simulink model "Test_of_GeneralForceCtro_VBS_Controller_tau_w"  (R2023a)
settings: Solver=FixedStepAuto  StartTime=0.0  StopTime=150  FixedStep=0.0001  RelTol=1e-3
libraries: simulink x2
settings Model: Creator=邓宇飞  LastModifiedBy=邓宇飞

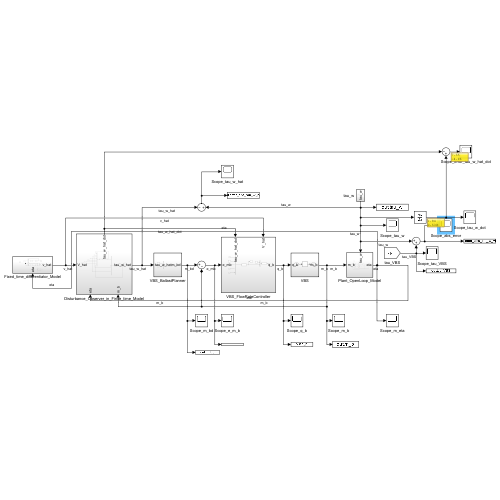
[thumbnail: Simulink's stored preview of the top-level diagram]
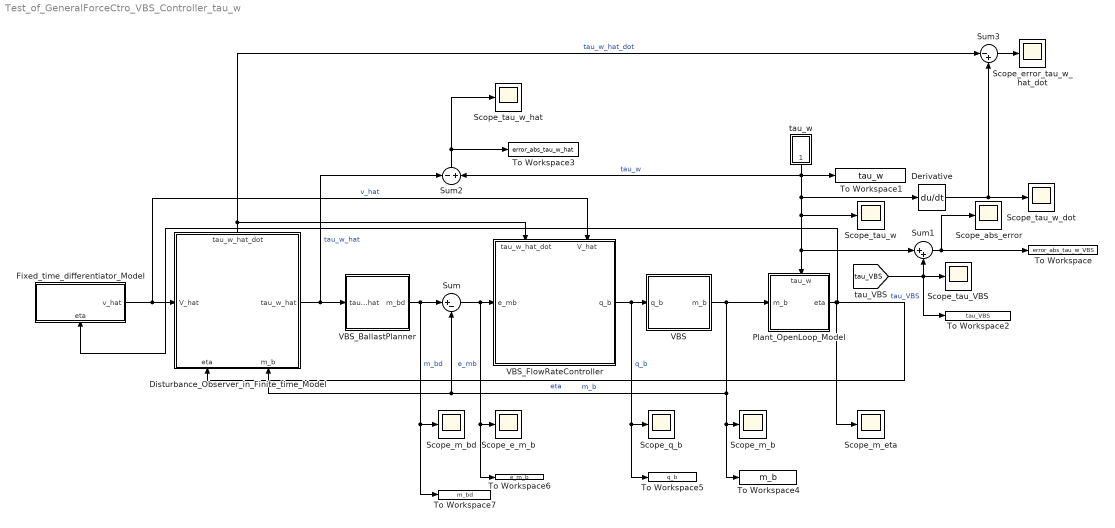
== system Test_of_GeneralForceCtro_VBS_Controller_tau_w ==
  Derivative : Derivative
  Disturbance_Observer_in_Finite_time_Model : Subsystem
      settings: PortSchema="{\"entries\":[{\"content\":{\"sides\":[{\"content\":{\"connectorIds\":[\"In1\"]},\"type\":\"ConnectorPlacement.EquallySpacedRectSide\",\"uuid\":\"977a3149-1921-48fe-b96a-a4ad28c91371\"},{\"content\":{\"connectorIds\":[\"Out1\"],\"side\":\"RIGHT\"},\"type\":\"ConnectorPlacement.EquallySpacedRectSide\",\"uuid\":\"fff94096-65c1-4681-8bdf-eed371b61c52\"},{\"content\":{\"connectorIds\":[\"Out2\"],\"side\":\"TOP\"},\"type\":\"ConnectorPlacement.EquallySpacedRectSide\",\"uuid\":\"5bed714d-ab4b-433b-a946-feaea2816cb1\"},{\"content\":{\"connectorIds\":[\"In2\",\"In3\"],\"side\":\"BOTTOM\"},\"type\":\"ConnectorPlacement.EquallySpacedRectSide\",\"uuid\":\"4ad85521-d335-4ab1-88b6-9b8c0a3b2785\"}]},\"type\":\"ConnectorPlacement.EquallySpacedConnector\",\"uuid\":\"7c33b186-f768-465e-b799-f94ef9fdf411\"}],\"packageUris\":[\"http://schema.mathworks.com/mf0/Connector/R2020b\"],\"version\":\"1.0\"}"
  Fixed_time_differentiator_Model : Subsystem
      settings: PortSchema="{\"entries\":[{\"content\":{\"sides\":[{\"content\":{},\"type\":\"ConnectorPlacement.EquallySpacedRectSide\",\"uuid\":\"509b689f-cae1-4523-9372-2499bd3b7d9d\"},{\"content\":{\"connectorIds\":[\"Out1\"],\"side\":\"RIGHT\"},\"type\":\"ConnectorPlacement.EquallySpacedRectSide\",\"uuid\":\"a1df743b-e6a9-4451-86f2-27990c18dc24\"},{\"content\":{\"side\":\"TOP\"},\"type\":\"ConnectorPlacement.EquallySpacedRectSide\",\"uuid\":\"5149f091-ad88-4d80-a39f-36dd9d24fd7a\"},{\"content\":{\"connectorIds\":[\"In1\"],\"side\":\"BOTTOM\"},\"type\":\"ConnectorPlacement.EquallySpacedRectSide\",\"uuid\":\"b5eefe9f-7883-4d8e-a8af-dce689347657\"}]},\"type\":\"ConnectorPlacement.EquallySpacedConnector\",\"uuid\":\"61175d6f-7ec4-4947-9258-193f13282eb9\"}],\"packageUris\":[\"http://schema.mathworks.com/mf0/Connector/R2020b\"],\"version\":\"1.0\"}"
  Plant_OpenLoop_Model : Subsystem
      settings: PortSchema="{\"entries\":[{\"content\":{\"sides\":[{\"content\":{\"connectorIds\":[\"In1\"]},\"type\":\"ConnectorPlacement.EquallySpacedRectSide\",\"uuid\":\"171ab365-2c9c-477f-ab94-6e1b535ce398\"},{\"content\":{\"connectorIds\":[\"Out1\"],\"side\":\"RIGHT\"},\"type\":\"ConnectorPlacement.EquallySpacedRectSide\",\"uuid\":\"68d15153-0085-4baf-9515-c294b6b9b8eb\"},{\"content\":{\"connectorIds\":[\"In2\"],\"side\":\"TOP\"},\"type\":\"ConnectorPlacement.EquallySpacedRectSide\",\"uuid\":\"3f887e7e-8b06-4bf2-b39d-d49324deef58\"}]},\"type\":\"ConnectorPlacement.EquallySpacedConnector\",\"uuid\":\"a8f2799e-4d6b-4adf-9803-c3f607cd4a91\"}],\"packageUris\":[\"http://schema.mathworks.com/mf0/Connector/R2020b\"],\"version\":\"1.0\"}"
  Scope_abs_error : Scope
  Scope_e_m_b : Scope
  Scope_error_tau_w_hat_dot : Scope
  Scope_m_b : Scope
  Scope_m_bd : Scope
  Scope_m_eta : Scope
  Scope_q_b : Scope
  Scope_tau_VBS : Scope
  Scope_tau_w : Scope
  Scope_tau_w_dot : Scope
  Scope_tau_w_hat : Scope
  Sum : Sum  Inputs=|+-
  Sum1 : Sum  Inputs=|++
  Sum2 : Sum  Inputs=-|+
  Sum3 : Sum  Inputs=|-+
  To Workspace : ToWorkspace  VariableName=error_abs_tau_w_VBS  SaveFormat=Timeseries  SampleTime=-1
  To Workspace1 : ToWorkspace  VariableName=tau_w  SaveFormat=Timeseries  SampleTime=-1
  To Workspace2 : ToWorkspace  VariableName=tau_VBS  SaveFormat=Timeseries  SampleTime=-1
  To Workspace3 : ToWorkspace  VariableName=error_abs_tau_w_hat  SaveFormat=Timeseries  SampleTime=-1
  To Workspace4 : ToWorkspace  VariableName=m_b  SaveFormat=Timeseries  SampleTime=-1
  To Workspace5 : ToWorkspace  VariableName=q_b  SaveFormat=Timeseries  SampleTime=-1
  To Workspace6 : ToWorkspace  VariableName=e_m_b  SaveFormat=Timeseries  SampleTime=-1
  To Workspace7 : ToWorkspace  VariableName=m_bd  SaveFormat=Timeseries  SampleTime=-1
  VBS : Subsystem
  VBS_BallastPlanner : Subsystem
  VBS_FlowRateController : Subsystem
      settings: PortSchema="{\"entries\":[{\"content\":{\"sides\":[{\"content\":{\"connectorIds\":[\"In1\"]},\"type\":\"ConnectorPlacement.EquallySpacedRectSide\",\"uuid\":\"977a3149-1921-48fe-b96a-a4ad28c91371\"},{\"content\":{\"connectorIds\":[\"Out1\"],\"side\":\"RIGHT\"},\"type\":\"ConnectorPlacement.EquallySpacedRectSide\",\"uuid\":\"fff94096-65c1-4681-8bdf-eed371b61c52\"},{\"content\":{\"connectorIds\":[\"In2\",\"In3\"],\"side\":\"TOP\"},\"type\":\"ConnectorPlacement.EquallySpacedRectSide\",\"uuid\":\"5bed714d-ab4b-433b-a946-feaea2816cb1\"}]},\"type\":\"ConnectorPlacement.EquallySpacedConnector\",\"uuid\":\"7c33b186-f768-465e-b799-f94ef9fdf411\"}],\"packageUris\":[\"http://schema.mathworks.com/mf0/Connector/R2020b\"],\"version\":\"1.0\"}"
  tau_w : Subsystem
  wires:
  tau_w/1(tau_w) -> To Workspace1/1, Derivative/1, Plant_OpenLoop_Model/2(tau_w), Sum1/1, Scope_tau_w/1, Sum2/2  "tau_w"
  VBS/1(m_b) -> Disturbance_Observer_in_Finite_time_Model/3(m_b), Sum/2, To Workspace4/1, Scope_m_b/1, Plant_OpenLoop_Model/1(m_b)  "m_b"
  [tau_VBS] -> To Workspace2/1, Scope_tau_VBS/1, Sum1/2  "tau_VBS"
  Disturbance_Observer_in_Finite_time_Model/1(tau_w_hat) -> Sum2/1, VBS_BallastPlanner/1(tau_w_hat)  "tau_w_hat"
  Fixed_time_differentiator_Model/1(v_hat) -> VBS_FlowRateController/3(V_hat), Disturbance_Observer_in_Finite_time_Model/1(V_hat)  "v_hat"
  VBS_FlowRateController/1(q_b) -> To Workspace5/1, Scope_q_b/1, VBS/1(q_b)  "q_b"
  Disturbance_Observer_in_Finite_time_Model/2(tau_w_hat_dot) -> Sum3/1, VBS_FlowRateController/2(tau_w_hat_dot)  "tau_w_hat_dot"
  Sum1/1 -> To Workspace/1, Scope_abs_error/1
  Plant_OpenLoop_Model/1(eta) -> Fixed_time_differentiator_Model/1(eta), Disturbance_Observer_in_Finite_time_Model/2(eta), Scope_m_eta/1  "eta"
  VBS_BallastPlanner/1(m_bd) -> To Workspace7/1, Scope_m_bd/1, Sum/1  "m_bd"
  Sum/1 -> Scope_e_m_b/1, To Workspace6/1, VBS_FlowRateController/1(e_mb)  "e_mb"
  Sum2/1 -> Scope_tau_w_hat/1, To Workspace3/1
  Derivative/1 -> Scope_tau_w_dot/1, Sum3/2
  Sum3/1 -> Scope_error_tau_w_hat_dot/1

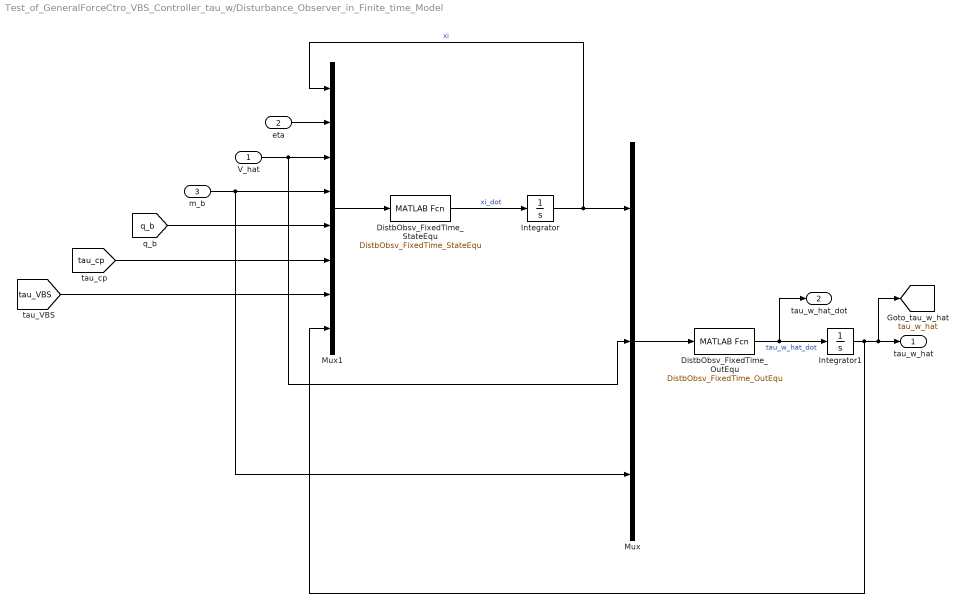
== system Test_of_GeneralForceCtro_VBS_Controller_tau_w/Disturbance_Observer_in_Finite_time_Model ==
  V_hat : Inport
  eta : Inport  Port=2
  m_b : Inport  Port=3
  DistbObsv_FixedTime_OutEqu : MATLABFcn  MATLABFcn=DistbObsv_FixedTime_OutEqu  OutputDimensions=2  OutputSignalType=real
  DistbObsv_FixedTime_StateEqu : MATLABFcn  MATLABFcn=DistbObsv_FixedTime_StateEqu  OutputDimensions=2  OutputSignalType=real
  Integrator : Integrator
  Integrator1 : Integrator
  Mux : Mux  Inputs=3
  Mux1 : Mux  Inputs=8
  tau_w_hat : Outport
  tau_w_hat_dot : Outport  Port=2
  tag scope: tau_w_hat=global
  wires:
  Integrator1/1 -> [tau_w_hat], tau_w_hat/1, Mux1/8
  Integrator/1 -> Mux1/1, Mux/1  "xi"
  DistbObsv_FixedTime_OutEqu/1 -> tau_w_hat_dot/1, Integrator1/1  "tau_w_hat_dot"
  Mux/1 -> DistbObsv_FixedTime_OutEqu/1
  Mux1/1 -> DistbObsv_FixedTime_StateEqu/1
  DistbObsv_FixedTime_StateEqu/1 -> Integrator/1  "xi_dot"
  eta/1 -> Mux1/2
  V_hat/1 -> Mux/2, Mux1/3
  m_b/1 -> Mux/3, Mux1/4
  [q_b] -> Mux1/5
  [tau_cp] -> Mux1/6
  [tau_VBS] -> Mux1/7

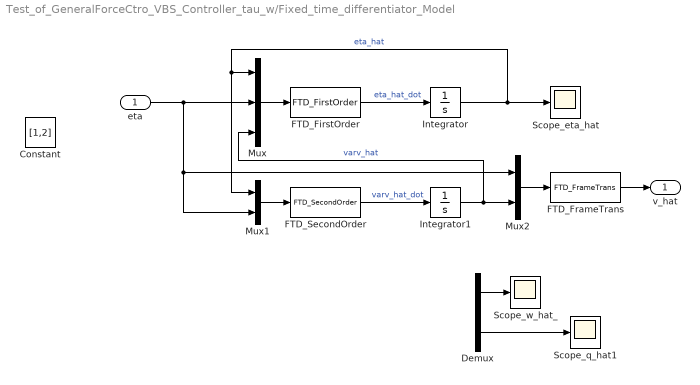
== system Test_of_GeneralForceCtro_VBS_Controller_tau_w/Fixed_time_differentiator_Model ==
  eta : Inport
  Constant : Constant  Value=[1,2]
  Demux : Demux  Outputs=2
  FTD_FirstOrder : MATLABFcn  MATLABFcn=FTD_FirstOrder  OutputDimensions=2
  FTD_FrameTrans : MATLABFcn  MATLABFcn=FTD_FrameTrans
  FTD_SecondOrder : MATLABFcn  MATLABFcn=FTD_SecondOrder  OutputDimensions=2
  Integrator : Integrator
  Integrator1 : Integrator
  Mux : Mux  Inputs=3
  Mux1 : Mux  Inputs=2
  Mux2 : Mux  Inputs=2
  Scope_eta_hat : Scope
  Scope_q_hat1 : Scope
  Scope_w_hat_ : Scope
  v_hat : Outport
  wires:
  Demux/1 -> Scope_w_hat_/1
  Integrator/1 -> Mux1/1, Mux/1, Scope_eta_hat/1  "eta_hat"
  Integrator1/1 -> Mux/3, Mux2/2  "varv_hat"
  Mux2/1 -> FTD_FrameTrans/1
  Mux/1 -> FTD_FirstOrder/1
  Mux1/1 -> FTD_SecondOrder/1
  Demux/2 -> Scope_q_hat1/1
  FTD_SecondOrder/1 -> Integrator1/1  "varv_hat_dot"
  FTD_FirstOrder/1 -> Integrator/1  "eta_hat_dot"
  eta/1 -> Mux2/1, Mux1/2, Mux/2
  FTD_FrameTrans/1 -> v_hat/1

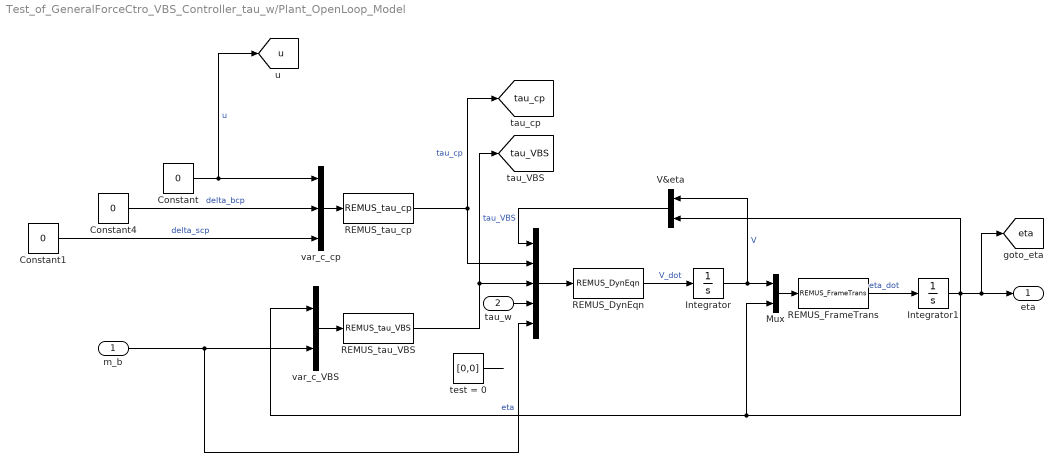
== system Test_of_GeneralForceCtro_VBS_Controller_tau_w/Plant_OpenLoop_Model ==
  m_b : Inport
  tau_w : Inport  Port=2
  " " : Mux  Inputs=5
  Constant : Constant  Value=0
  Constant1 : Constant  Value=0
  Constant4 : Constant  Value=0
  Integrator : Integrator
  Integrator1 : Integrator
  Mux : Mux  Inputs=2
  REMUS_DynEqn : MATLABFcn  MATLABFcn=REMUS_DynEqn  OutputDimensions=2
  REMUS_FrameTrans : MATLABFcn  MATLABFcn=REMUS_FrameTrans  OutputDimensions=2
  REMUS_tau_VBS : MATLABFcn  MATLABFcn=REMUS_tau_VBS  OutputDimensions=2  OutputSignalType=real
  REMUS_tau_cp : MATLABFcn  MATLABFcn=REMUS_tau_cp  OutputDimensions=2  OutputSignalType=real
  V&eta : Mux  Inputs=2
  test = 0 : Constant  Value=[0,0]
  var_c_VBS : Mux  Inputs=2
  var_c_cp : Mux  Inputs=3
  eta : Outport
  tag scope: eta=global, tau_VBS=global, tau_cp=global, u=global
  wires:
  Constant/1 -> [u], var_c_cp/1  "u"
  REMUS_DynEqn/1 -> Integrator/1  "V_dot"
  REMUS_tau_cp/1 -> [tau_cp], " "/2  "tau_cp"
  Integrator1/1 -> [eta], eta/1, Mux/2, var_c_VBS/1, V&eta/2  "eta"
  Constant1/1 -> var_c_cp/3  "delta_scp"
  test = 0/1 -> ?
  Mux/1 -> REMUS_FrameTrans/1
  " "/1 -> REMUS_DynEqn/1
  Integrator/1 -> Mux/1, V&eta/1  "V"
  Constant4/1 -> var_c_cp/2  "delta_bcp"
  var_c_cp/1 -> REMUS_tau_cp/1
  V&eta/1 -> " "/1
  REMUS_tau_VBS/1 -> [tau_VBS], " "/3  "tau_VBS"
  tau_w/1 -> " "/4
  REMUS_FrameTrans/1 -> Integrator1/1  "eta_dot"
  var_c_VBS/1 -> REMUS_tau_VBS/1
  m_b/1 -> " "/5, var_c_VBS/2

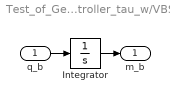
== system Test_of_GeneralForceCtro_VBS_Controller_tau_w/VBS ==
  q_b : Inport
  Integrator : Integrator
  m_b : Outport
  wires:
  q_b/1 -> Integrator/1
  Integrator/1 -> m_b/1

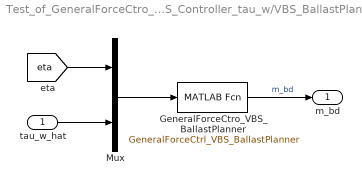
== system Test_of_GeneralForceCtro_VBS_Controller_tau_w/VBS_BallastPlanner ==
  tau_w_hat : Inport
  GeneralForceCtro_VBS_BallastPlanner : MATLABFcn  MATLABFcn=GeneralForceCtrl_VBS_BallastPlanner  OutputDimensions=2  OutputSignalType=real
  Mux : Mux  Inputs=2
  m_bd : Outport
  wires:
  Mux/1 -> GeneralForceCtro_VBS_BallastPlanner/1
  GeneralForceCtro_VBS_BallastPlanner/1 -> m_bd/1  "m_bd"
  [eta] -> Mux/1
  tau_w_hat/1 -> Mux/2

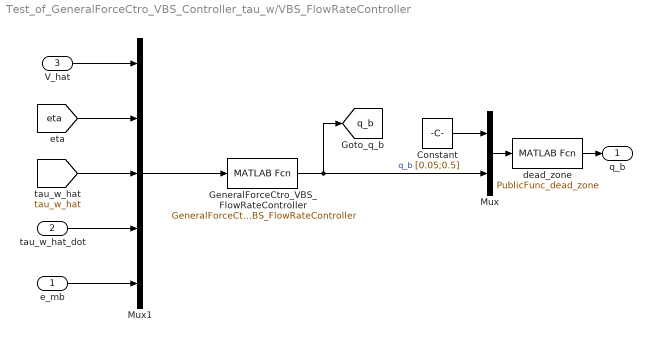
== system Test_of_GeneralForceCtro_VBS_Controller_tau_w/VBS_FlowRateController ==
  e_mb : Inport
  tau_w_hat_dot : Inport  Port=2
  V_hat : Inport  Port=3
  Constant : Constant  Value=[0.05;0.5]
  GeneralForceCtro_VBS_FlowRateController : MATLABFcn  MATLABFcn=GeneralForceCtrl_VBS_FlowRateController  OutputDimensions=2  OutputSignalType=real
  Mux : Mux  Inputs=2
  Mux1 : Mux  Inputs=5
  dead_zone : MATLABFcn  MATLABFcn=PublicFunc_dead_zone  OutputDimensions=2  OutputSignalType=real
  q_b : Outport
  tag scope: q_b=global
  wires:
  Mux1/1 -> GeneralForceCtro_VBS_FlowRateController/1
  GeneralForceCtro_VBS_FlowRateController/1 -> Mux/2, [q_b]  "q_b"
  V_hat/1 -> Mux1/1
  [eta] -> Mux1/2
  [tau_w_hat] -> Mux1/3
  tau_w_hat_dot/1 -> Mux1/4
  e_mb/1 -> Mux1/5
  dead_zone/1 -> q_b/1
  Mux/1 -> dead_zone/1
  Constant/1 -> Mux/1

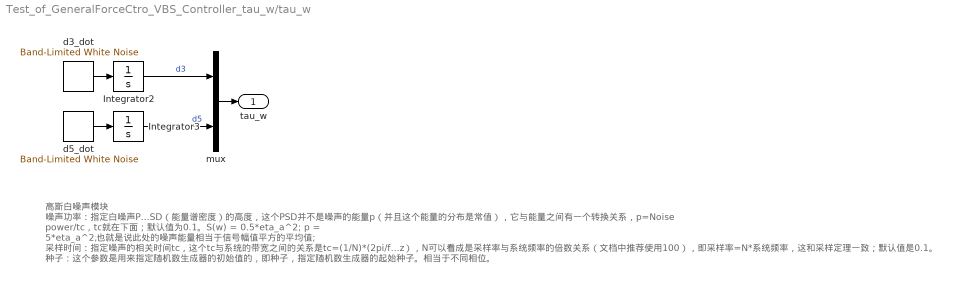
== system Test_of_GeneralForceCtro_VBS_Controller_tau_w/tau_w ==
  note: 高斯白噪声模块
      | 噪声功率：指定白噪声PSD（能量谱密度）的高度，这个PSD并不是噪声的能量p（并且这个能量的分布是常值），它与能量之间有一个转换关系，p=Noise power/tc，tc就在下面；默认值为0.1。S(w) = 0.5*eta_a^2;
      | p = 5*eta_a^2;也就是说此处的噪声能量相当于信号幅值平方的平均值;
      | 采样时间：指定噪声的相关时间tc，这个tc与系统的带宽之间的关系是tc=(1/N)*(2pi/fmax)，其中fmax是系统的带宽（实际上是角频率，fmax=2*pi*f，这个f才是我们常使用的频率Hz），N可以看成是采样率与系统频率的倍数关系（文档中推荐使用100），即采样率=N*系统频率，这和采样定理一致；默认值是0.1。
      | 种子：这个参数是用来指定随机数生成器的初始值的，即种子，指定随机数生成器的起始种子。相当于不同相位。
  Integrator2 : Integrator
  Integrator3 : Integrator
  d3_dot : simulink/Sources/Band-Limited White Noise  Cov=[0.5]  Ts=0.1  seed=[2]
  d5_dot : simulink/Sources/Band-Limited White Noise  Cov=[0.1]  Ts=0.1  seed=[3]
  mux : Mux  Inputs=2
  tau_w : Outport
  wires:
  Integrator3/1 -> mux/2  "d5"
  d5_dot/1 -> Integrator3/1
  d3_dot/1 -> Integrator2/1
  mux/1 -> tau_w/1
  Integrator2/1 -> mux/1  "d3"
